simulink model "dsrc_utils"  (Simulink 8.2)
settings: Solver=ode1  StartTime=0.0  StopTime=Inf  FixedStep=0.001  RelTol=1e-3
PostLoadFcn:
  | , if any(exist('dsrtsu_mdlpostloadfcn', 'file') == [2, 3, 6]), try dsrtsu_mdlpostloadfcn('Execute', bdroot); catch fprintf('Error in PostLoadFcn (dsrtsu_mdlpostloadfcn) for model "%s":\n %s\n', bdroot, lasterr); end, end,
settings Model: DSRTSU_INTERNAL_RTI_VER=450  DSRTSU_INTERNAL_RTI_TYPE=rti1401  DSRTSU_INTERNAL_RTIFPGA=40  Creator=rushk1  LastModifiedBy=rushk1  BufferReuse=off
settings DataIOCC: SignalLoggingSaveFormat=Dataset
settings OptimizationCC: BlockReduction=off  OptimizeBlockIOStorage=off  BufferReuse=off  ExpressionFolding=off  ExpressionDepthLimit=128  LocalBlockOutputs=off
settings DebuggingCC: FcnCallInpInsideContextMsg=EnableAllAsError  StateNameClashWarn=none
settings HardwareCC: TargetHWDeviceType=Generic->Custom
settings RTWCC: SystemTargetFile=rti1401.tlc  MakeCommand=make_rti  TemplateMakefile=rti1401.tmf  Description=dSPACE DS1401 Hardware Platform  ProcessScript=rti1401_make_rtw_hook
settings STFCustomTargetCC: CodeReplacementLibrary=ANSI_C  ParMdlRefBuildCompliant=on  GeneratePreprocessorConditionals=Disable all  MatFileLogging=on  SystemTargetFile=rti1401.tlc
settings GRTTargetCC: CompOptLevelCompliant=off  ConcurrentExecutionCompliant=off  ExtModeMexFile=noextcomm
settings CustomProperty: DataType=RTWOptions_EnumType_C__Program Files_dSPACE RCPHIL 2014-B_MATLAB_RTI_RTI1401_TLC_rti1401_1InitialSimState  Value=RUN
settings EnumStrPairs: String=RUN

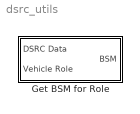
== system dsrc_utils ==
  Get BSM for Role : Subsystem

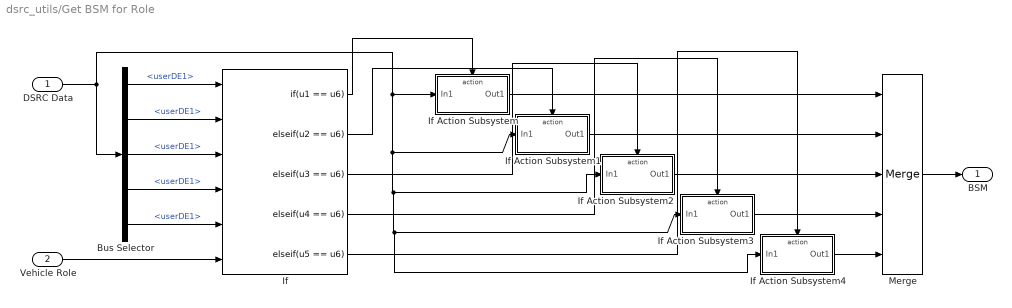
== system dsrc_utils/Get BSM for Role ==
  DSRC Data : Inport  OutDataTypeStr=Bus: BSMStoreBus
  Vehicle Role : Inport  Port=2  OutDataTypeStr=Enum: VehicleRoleEnum
  Bus Selector : BusSelector  OutputSignals=Veh1BSM.userDE1,Veh2BSM.userDE1,Veh3BSM.userDE1,Veh4BSM.userDE1,Veh5BSM.userDE1
  If : If  NumInputs=6  IfExpression=u1 == u6  ElseIfExpressions=u2 == u6,u3 == u6, u4 == u6, u5 == u6  ShowElse=off
  If Action Subsystem : Subsystem  TreatAsAtomicUnit=on
  If Action Subsystem1 : Subsystem  TreatAsAtomicUnit=on
  If Action Subsystem2 : Subsystem  TreatAsAtomicUnit=on
  If Action Subsystem3 : Subsystem  TreatAsAtomicUnit=on
  If Action Subsystem4 : Subsystem  TreatAsAtomicUnit=on
  Merge : Merge  Inputs=5
  BSM : Outport
  wires:
  DSRC Data/1 -> Bus Selector/1, If Action Subsystem4/1(In1), If Action Subsystem3/1(In1), If Action Subsystem2/1(In1), If Action Subsystem1/1(In1), If Action Subsystem/1(In1)
  Bus Selector/1 -> If/1  "<userDE1>"
  Bus Selector/4 -> If/4  "<userDE1>"
  Bus Selector/5 -> If/5  "<userDE1>"
  Bus Selector/3 -> If/3  "<userDE1>"
  Bus Selector/2 -> If/2  "<userDE1>"
  Vehicle Role/1 -> If/6
  If/1 -> If Action Subsystem/Action
  If/2 -> If Action Subsystem1/Action
  If/3 -> If Action Subsystem2/Action
  If/4 -> If Action Subsystem3/Action
  If/5 -> If Action Subsystem4/Action
  If Action Subsystem4/1(Out1) -> Merge/5
  If Action Subsystem3/1(Out1) -> Merge/4
  If Action Subsystem2/1(Out1) -> Merge/3
  If Action Subsystem1/1(Out1) -> Merge/2
  If Action Subsystem/1(Out1) -> Merge/1
  Merge/1 -> BSM/1

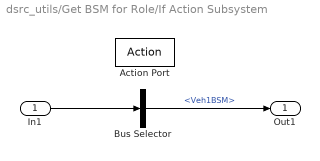
== system dsrc_utils/Get BSM for Role/If Action Subsystem ==
  In1 : Inport
  Action Port : ActionPort  ActionType=then
  Bus Selector : BusSelector  OutputSignals=Veh1BSM
  Out1 : Outport
  wires:
  In1/1 -> Bus Selector/1
  Bus Selector/1 -> Out1/1  "<Veh1BSM>"

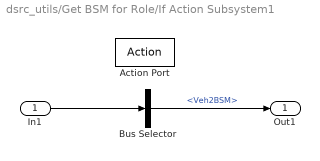
== system dsrc_utils/Get BSM for Role/If Action Subsystem1 ==
  In1 : Inport
  Action Port : ActionPort  ActionType=elseif
  Bus Selector : BusSelector  OutputSignals=Veh2BSM
  Out1 : Outport
  wires:
  In1/1 -> Bus Selector/1
  Bus Selector/1 -> Out1/1  "<Veh2BSM>"

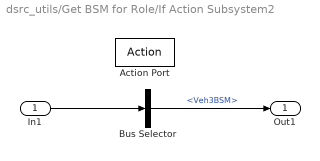
== system dsrc_utils/Get BSM for Role/If Action Subsystem2 ==
  In1 : Inport
  Action Port : ActionPort  ActionType=elseif
  Bus Selector : BusSelector  OutputSignals=Veh3BSM
  Out1 : Outport
  wires:
  In1/1 -> Bus Selector/1
  Bus Selector/1 -> Out1/1  "<Veh3BSM>"

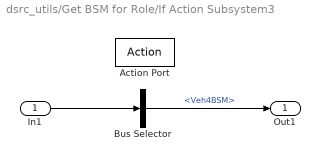
== system dsrc_utils/Get BSM for Role/If Action Subsystem3 ==
  In1 : Inport
  Action Port : ActionPort  ActionType=elseif
  Bus Selector : BusSelector  OutputSignals=Veh4BSM
  Out1 : Outport
  wires:
  In1/1 -> Bus Selector/1
  Bus Selector/1 -> Out1/1  "<Veh4BSM>"

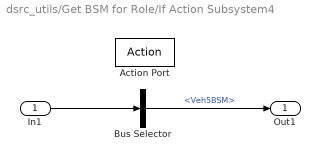
== system dsrc_utils/Get BSM for Role/If Action Subsystem4 ==
  In1 : Inport
  Action Port : ActionPort  ActionType=elseif
  Bus Selector : BusSelector  OutputSignals=Veh5BSM
  Out1 : Outport
  wires:
  In1/1 -> Bus Selector/1
  Bus Selector/1 -> Out1/1  "<Veh5BSM>"
